simulink model "testing_sim_func"  (R2019b)
settings: Solver=VariableStepAuto  StartTime=0.0  StopTime=10.0  RelTol=1e-3
settings Model: Creator=arund  LastModifiedBy=arund

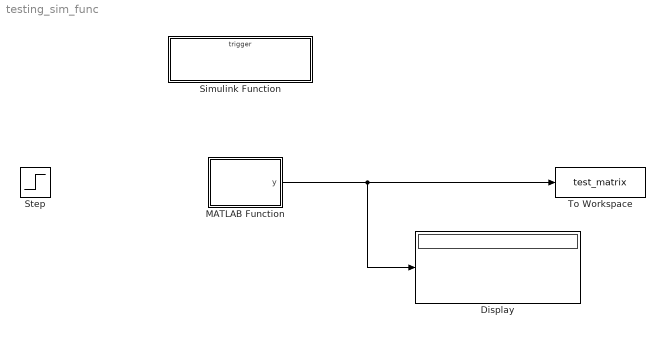
== system testing_sim_func ==
  Display : Display
  MATLAB Function : MATLAB Function  TreatAsAtomicUnit=on
  Simulink Function : Subsystem  TreatAsAtomicUnit=on
  Step : Step  SampleTime=0
  To Workspace : ToWorkspace  VariableName=test_matrix  SaveFormat=Timeseries  SampleTime=-1
  wires:
  MATLAB Function/1(y) -> Display/1, To Workspace/1

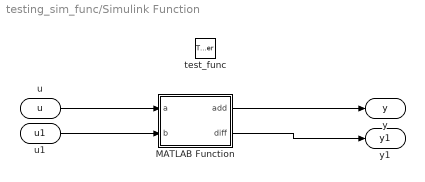
== system testing_sim_func/Simulink Function ==
  test_func : TriggerPort  TriggerType=function-call  IsSimulinkFunction=on  FunctionName=test_func  FunctionVisibility=scoped  VariantControl=(inherit)
  MATLAB Function : MATLAB Function  TreatAsAtomicUnit=on
  u : ArgIn  DisableCoverage=on  ArgumentName=u
  u1 : ArgIn  DisableCoverage=on  Port=2  ArgumentName=u1
  y : ArgOut  DisableCoverage=on  ArgumentName=y
  y1 : ArgOut  DisableCoverage=on  Port=2  ArgumentName=y1
  wires:
  u/1 -> MATLAB Function/1(a)
  MATLAB Function/1(add) -> y/1
  MATLAB Function/2(diff) -> y1/1
  u1/1 -> MATLAB Function/2(b)

== matlab function testing_sim_func/MATLAB Function ==
  data: y output
function y = fcn()
[ans1 ans2]=test_func(3,2);
y=[ans1 ans2];

== matlab function testing_sim_func/Simulink Function/MATLAB Function ==
  data: a input; add output; b input; diff output
function [add,diff]  = fcn(a,b)

add=a+b;
diff=a-b
